simulink model "F_7"  (R2017a)
settings: Solver=ode45  StartTime=0.0  StopTime=50  MaxStep=.1  RelTol=1e-3  EnableMultiTasking=on
InitFcn:
  | addpath ./..
  | F_param
undefined symbols (not defined in the file or in its folder): F_animation
libraries: simulink x3
settings Model: Creator=beard  LastModifiedBy=Mat Haskell
settings DataIOCC: LimitDataPoints=on  SaveFormat=Array  SignalLoggingSaveFormat=ModelDataLogs
settings OptimizationCC: ExpressionDepthLimit=2147483647  InitFltsAndDblsToZero=on  LifeSpan=inf
settings DebuggingCC: UnderspecifiedInitializationDetection=Classic  MergeDetectMultiDrivingBlocksExec=none  SolverPrmCheckMsg=warning  FcnCallInpInsideContextMsg=warning  StateNameClashWarn=warning  SFUnexpectedBacktrackingDiag=warning  SFNoUnconditionalDefaultTransitionDiag=warning  SFExecutionAtInitializationDiag=none
settings HardwareCC: ProdBitPerPointer=32  ProdBitPerSizeT=32  ProdBitPerPtrDiffT=32  ProdLargestAtomicFloat=None  ProdIntDivRoundTo=Undefined  ProdEndianess=Unspecified  ProdWordSize=32  ProdHWDeviceType=32-bit Generic
settings ModelReferenceCC: PropagateSignalLabelsOutOfModel=off
settings GRTTargetCC: TargetLangStandard=C89/C90 (ANSI)  GeneratePreprocessorConditionals=Disable all  CombineOutputUpdateFcns=off  GRTInterface=on
settings ConfigComp: CovMetricSettings=dw  CovHtmlReporting=on  CovSaveCumulativeToWorkspaceVar=on  CovSaveSingleToWorkspaceVar=on  CovExternalEMLEnable=off

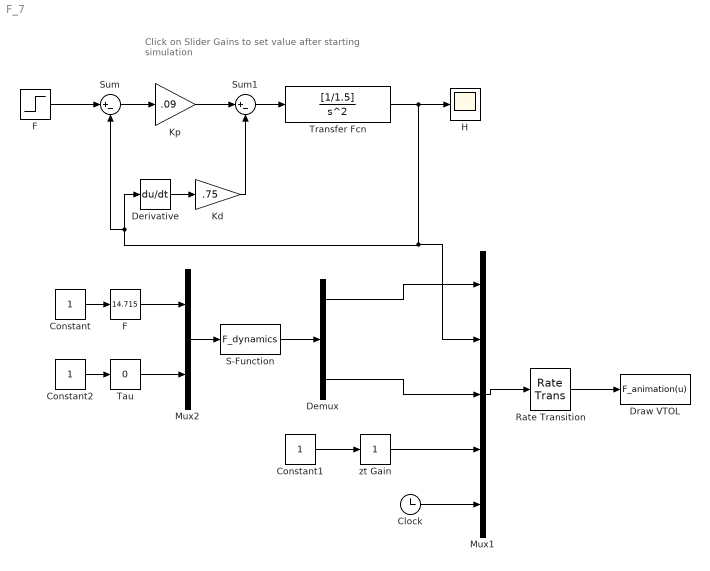
== system F_7 ==
  note: Click on Slider Gains to set value
      | after starting simulation
  Clock : Clock
  Constant : Constant
  Constant1 : Constant
  Constant2 : Constant
  Demux : Demux  Outputs=3
  Derivative : Derivative
  Draw VTOL : MATLABFcn  InitFcn=|  MATLABFcn=F_animation(u)  OutputDimensions=0
      | clear;clc
      | F_param
  F : simulink/Math Operations/Slider Gain  gain=14.715  low=0  high=20
  "F " : Step  SampleTime=0
  "H " : Scope
  "Kd " : Gain  Gain=.75
  Kp : Gain  Gain=.09
  Mux1 : Mux  Inputs=5
  Mux2 : Mux  Inputs=2
  Rate Transition : RateTransition  OutPortSampleTime=P.t_plot
  S-Function : S-Function  FunctionName=F_dynamics  Parameters=P  SFunctionDeploymentMode=off  EnableBusSupport=off
  Sum : Sum  Inputs=|+-
  Sum1 : Sum  Inputs=|+-
  Tau : simulink/Math Operations/Slider Gain  gain=0  low=-2  high=2
  Transfer Fcn : TransferFcn  Numerator=[1/1.5]  Denominator=[1 0 0]
  zt Gain : simulink/Math Operations/Slider Gain  gain=1  low=0  high=5
  wires:
  Mux1/1 -> Rate Transition/1
  Rate Transition/1 -> Draw VTOL/1
  Constant/1 -> F/1
  Constant1/1 -> zt Gain/1
  Mux2/1 -> S-Function/1
  F/1 -> Mux2/1
  Tau/1 -> Mux2/2
  Constant2/1 -> Tau/1
  Derivative/1 -> "Kd "/1
  Sum/1 -> Kp/1
  Transfer Fcn/1 -> Mux1/2, Sum/2, Derivative/1, "H "/1
  "Kd "/1 -> Sum1/2
  Sum1/1 -> Transfer Fcn/1
  Kp/1 -> Sum1/1
  "F "/1 -> Sum/1
  S-Function/1 -> Demux/1
  Clock/1 -> Mux1/5
  zt Gain/1 -> Mux1/4
  Demux/3 -> Mux1/3
  Demux/1 -> Mux1/1
